simulink model "sf_elevator_old"  (R2017b)
settings: Solver=FixedStepDiscrete  StartTime=0.0  StopTime=inf  FixedStep=0.01  RelTol=1e-3  EnableMultiTasking=on
InitFcn:
  | allCarIds = [1 2];
StartFcn:
  | sf_elevator_gui('init', 'sf_elevator_old', allCarIds);
StopFcn:
  | sf_elevator_gui('close');
CloseFcn:
  | sf_elevator_gui('close');
  | clear allCarIds;
settings Model: ExtModeAutoUpdateStatusClock=off  Creator=The MathWorks, Inc.  LastModifiedBy=The MathWorks, Inc.
settings DataIOCC: LimitDataPoints=on  SaveFormat=StructureWithTime  SignalLoggingName=sigsOut
settings OptimizationCC: ExpressionDepthLimit=2147483647  InitFltsAndDblsToZero=on  EfficientMapNaN2IntZero=off  LifeSpan=Inf
settings DebuggingCC: SaveWithParameterizedLinksMsg=none  UnderspecifiedInitializationDetection=Classic  MergeDetectMultiDrivingBlocksExec=none  MultiTaskDSMMsg=warning  MultiTaskCondExecSysMsg=none  MultiTaskRateTransMsg=warning  FcnCallInpInsideContextMsg=warning  StateNameClashWarn=warning  StrictBusMsg=None  SFUnexpectedBacktrackingDiag=warning  SFNoUnconditionalDefaultTransitionDiag=warning  SFExecutionAtInitializationDiag=none
settings HardwareCC: ProdBitPerPointer=32  ProdBitPerSizeT=32  ProdBitPerPtrDiffT=32  ProdLargestAtomicFloat=None  ProdIntDivRoundTo=Undefined  ProdEndianess=Unspecified  ProdWordSize=32  ProdHWDeviceType=32-bit Generic  TargetUnknown=on
settings ModelReferenceCC: PropagateSignalLabelsOutOfModel=off
settings SFSimCC: SFSimEcho=off  SimIntegrity=off  SimParseCustomCode=off  MATLABDynamicMemAlloc=off
settings RTWCC: SystemTargetFile=ert.tlc  TemplateMakefile=ert_default_tmf  Description=Real-Time Workshop Embedded Coder
settings CodeAppCC: IgnoreCustomStorageClasses=off  CustomSymbolStrType=$N$R$M  StateflowObjectComments=on  InternalIdentifier=Classic
settings ERTTargetCC: MultiwordLength=2048  GenerateSampleERTMain=on  ERTCustomFileTemplate=example_file_process.tlc  ConvertIfToSwitch=off  SuppressUnreachableDefaultCases=off
settings ConfigComp: CovMetricSettings=dcmtr  CovHtmlReporting=on  CovSaveCumulativeToWorkspaceVar=on  CovSaveSingleToWorkspaceVar=on  CovExternalEMLEnable=off  CovSFcnEnable=off

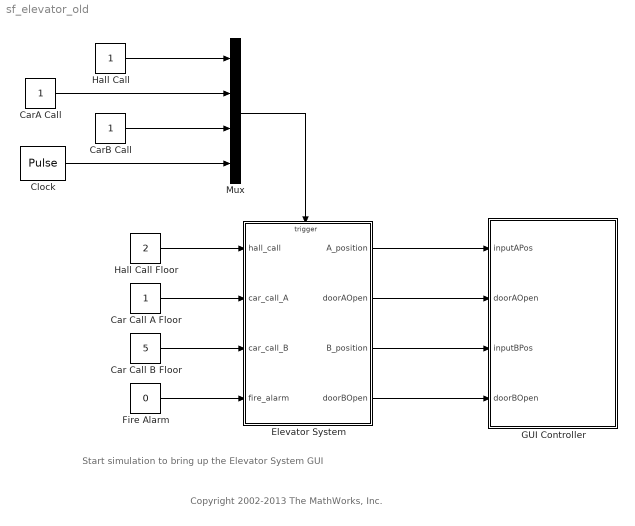
== system sf_elevator_old ==
  note: Start simulation to bring up the Elevator System GUI
  note: Copyright 2002-2013 The MathWorks, Inc.
  Car Call A Floor : Constant  OutDataTypeStr=uint8
  Car Call B Floor : Constant  Value=5  OutDataTypeStr=uint8
  CarA Call : Constant  OutDataTypeStr=double
  CarB Call : Constant  OutDataTypeStr=double
  Clock : DiscretePulseGenerator  PulseType=Time based  PulseWidth=50
  Elevator System : Stateflow chart  TreatAsAtomicUnit=on
  Fire Alarm : Constant  Value=0  OutDataTypeStr=uint8
  GUI Controller : Stateflow chart  TreatAsAtomicUnit=on
  Hall Call : Constant  OutDataTypeStr=double
  Hall Call Floor : Constant  Value=2  OutDataTypeStr=uint8
  Mux : Mux
  wires:
  Hall Call Floor/1 -> Elevator System/1(hall_call)
  Car Call A Floor/1 -> Elevator System/2(car_call_A)
  Car Call B Floor/1 -> Elevator System/3(car_call_B)
  Fire Alarm/1 -> Elevator System/4(fire_alarm)
  Hall Call/1 -> Mux/1
  CarA Call/1 -> Mux/2
  CarB Call/1 -> Mux/3
  Clock/1 -> Mux/4
  Mux/1 -> Elevator System/Trigger
  Elevator System/1(A_position) -> GUI Controller/1(inputAPos)
  Elevator System/2(doorAOpen) -> GUI Controller/2(doorAOpen)
  Elevator System/3(B_position) -> GUI Controller/3(inputBPos)
  Elevator System/4(doorBOpen) -> GUI Controller/4(doorBOpen)

== stateflow chart sf_elevator_old/Elevator System ==
  state Elevator_Manager [parallel]
    du: A_position = Elevator_A.get_position();
    B_position = Elevator_B.get_position();
    settings: executionOrder=1
    state process_hall_call() [function]
      (default) -> (junction 1685)
      (junction 1685) -> (junction 1687) : {
          | /* 'INIT':Initialization */
          | request_floor = hall_call_queue[0];
          | }
      (junction 1687) -> (junction 1689) : {
          | /* Fire alarm is on */
          | fire_alarm_on = (fire_alarm);
          | }
      (junction 1689) -> (junction 1691) : {
          | /* There is outstanding request */
          | request_outstanding = (request_floor > 0);
          | }
      (junction 1691) -> (junction 1693) : {
          | /* Elevator A is idle */
          | elevator_A_idle = (Elevator_A.get_status() == IDLE);
          | }
      (junction 1693) -> (junction 1695) : {
          | /* Elevator B is idle */
          | elevator_B_idle = (Elevator_B.get_status() == IDLE);
          | }
      (junction 1695) -> (junction 1697) : {
          | /* Elevator A is closer to request */
          | elevator_A_closer = (fabs(Elevator_A.get_position() - request_floor) <= fabs(Elevator_B.get_position() - request_floor));
          | }
      (junction 1697) -> (junction 1699) [order 1] : [fire_alarm_on]
      (junction 1699) -> (junction 1701) : {
          | /* 'EMR':Emergency */
          | Elevator_A.register(floor(Elevator_A.get_position()+Elevator_A.get_direction()/2));
          | Elevator_B.register(floor(Elevator_B.get_position()+Elevator_B.get_direction()/2));
          | }
      (junction 1697) -> (junction 1703) [order 2]
      (junction 1703) -> (junction 1705) [order 1] : [!request_outstanding]
      (junction 1705) -> (junction 1707) : {
          | /* 'NONE':Both elevators are busy or no request present */
          |
          | }
      (junction 1703) -> (junction 1709) [order 2]
      (junction 1709) -> (junction 1711) [order 1] : [!elevator_A_idle && !elevator_B_idle]
      (junction 1711) -> (junction 1713) : {
          | /* 'NONE':Both elevators are busy or no request present */
          |
          | }
      (junction 1709) -> (junction 1715) [order 2]
      (junction 1715) -> (junction 1717) [order 1] : [elevator_A_idle && !elevator_B_idle]
      (junction 1717) -> (junction 1719) : {
          | /* 'A':Elevator A should respond to request */
          | Elevator_A.enqueue(request_floor);
          | dequeue(request_floor);
          | }
      (junction 1715) -> (junction 1721) [order 2]
      (junction 1721) -> (junction 1723) [order 1] : [!elevator_A_idle && elevator_B_idle]
      (junction 1723) -> (junction 1725) : {
          | /* 'B':Elevator B should respond to request */
          | Elevator_B.enqueue(request_floor);
          | dequeue(request_floor);
          | }
      (junction 1721) -> (junction 1727) [order 2]
      (junction 1727) -> (junction 1729) [order 1] : [elevator_A_idle && elevator_B_idle && elevator_A_closer]
      (junction 1729) -> (junction 1731) : {
          | /* 'A':Elevator A should respond to request */
          | Elevator_A.enqueue(request_floor);
          | dequeue(request_floor);
          | }
      (junction 1727) -> (junction 1733) [order 2]
      (junction 1733) -> (junction 1735) [order 1] : [elevator_A_idle && elevator_B_idle && !elevator_A_closer]
      (junction 1735) -> (junction 1737) : {
          | /* 'B':Elevator B should respond to request */
          | Elevator_B.enqueue(request_floor);
          | dequeue(request_floor);
          | }
      (junction 1733) -> (junction 1739) [order 2]
    state ans = exists_in_queue(floor) [function]
      (default) -> (junction 304) : {i=0;}
      (junction 304) -> (junction 304) [order 1] : [hall_call_queue[i] > 0 && ...
          | i<NUM_FLOOR && ...
          | hall_call_queue[i] != floor]{i++;}
      (junction 304) -> (junction 303) [order 2]
      (junction 303) -> (junction 302) [order 1] : [i >= NUM_FLOOR || hall_call_queue[i] == 0]{ans = 0;}
      (junction 303) -> (junction 301) [order 2] : {ans = i+1;}
    state register(hall_call_floor) [function]
      (default) -> (junction 269) : {enqueue(hall_call_floor);
          | hall_call_status[hall_call_floor] = 1;}
    state deregister(hall_call_floor) [function]
      (default) -> (junction 272) : {dequeue(hall_call_floor);
          | hall_call_status[hall_call_floor] = 0;}
    state enqueue(hall_call_floor) [function]
      (default) -> (junction 217)
      (junction 217) -> (junction 216) [order 1] : [hall_call_status[hall_call_floor] != 0]
      (junction 217) -> (junction 234) [order 2] : {i = 0;}
      (junction 234) -> (junction 233) [order 1] : [hall_call_queue[i] == hall_call_floor]
      (junction 234) -> (junction 234) [order 2] : [hall_call_queue[i] > 0 && i<NUM_FLOOR]{i++;}
      (junction 234) -> (junction 232) [order 3]
      (junction 232) -> (junction 227) [order 1] : [i >= NUM_FLOOR]
      (junction 232) -> (junction 228) [order 2] : {hall_call_queue[i] = hall_call_floor;}
    state dequeue(hall_call_floor) [function]
      (default) -> (junction 231) : {i=0;}
      (junction 231) -> (junction 231) [order 1] : [hall_call_queue[i] > 0 && ...
          | i<NUM_FLOOR && ...
          | hall_call_queue[i] != hall_call_floor]{i++;}
      (junction 231) -> (junction 212) [order 2]
      (junction 212) -> (junction 211) [order 1] : [i >= NUM_FLOOR || hall_call_queue[i] == 0]
      (junction 212) -> (junction 206) [order 2]
      (junction 206) -> (junction 230) : {hall_call_queue[i] = hall_call_queue[i+1]; i++;}
      (junction 230) -> (junction 206) [order 1] : [i < NUM_FLOOR]
      (junction 230) -> (junction 274) [order 2]
    Elevator_Manager -> (junction 229) [order 1] : HALL_CALL{register(hall_call);}
    Elevator_Manager -> (junction 1430) [order 2] : CLOCK {process_hall_call();}
  state Elevator_B [parallel]
    settings: executionOrder=3
    state PickUpDropOff
      en: Elevator_Manager.deregister(cur_floor);
      deregister(cur_floor);
      direction = MOVE_IDLE;
      doorBOpen = 1;
      du: Elevator_Manager.deregister(cur_floor);
      deregister(cur_floor);
      ex: doorBOpen = 0;
      state Stopped
      Elevator_B.PickUpDropOff.Stopped -> Elevator_B.PickUpDropOff.Stopped [order 2] : [fire_alarm]{status = EMERG;}
          | /* Resets the timeout counter */
    state Idle
      en: status = IDLE;
      ex: status = BUSY;
    state MoveToTask
      du: move_to(task_queue[0]);
    state move_to(destination) [function]
      (default) -> (junction 1615)
      (junction 1615) -> (junction 1617) : {
          | /* Move up */
          | move_up = (destination - position > ERR_TOR);
          | }
      (junction 1617) -> (junction 1619) : {
          | /* Move down */
          | move_down = (position - destination > ERR_TOR);
          | }
      (junction 1619) -> (junction 1621) [order 1] : [move_up && !move_down]
      (junction 1621) -> (junction 1623) : {
          | /* Move up */
          | position = position + VELOCITY;
          | direction = MOVE_UP;
          | }
      (junction 1619) -> (junction 1625) [order 2]
      (junction 1625) -> (junction 1627) [order 1] : [!move_up && move_down]
      (junction 1627) -> (junction 1629) : {
          | /* Move down */
          | position = position - VELOCITY;
          | direction = MOVE_DOWN;
          | }
      (junction 1625) -> (junction 1631) [order 2]
    state ans = should_stop [function]
      (default) -> (junction 1638)
      (junction 1638) -> (junction 1640) : {
          | /* 'INIT':Initialization */
          | cur_floor = ml_round(position);
          | }
      (junction 1640) -> (junction 1642) : {
          | /* Arrived destination */
          | at_destination = (fabs(position - task_queue[0]) < ERR_TOR);
          | }
      (junction 1642) -> (junction 1644) : {
          | /* Arrived a floor */
          | at_a_floor = (fabs(position - cur_floor) < ERR_TOR);
          | }
      (junction 1644) -> (junction 1646) : {
          | /* There is car call to stop at this floor */
          | request_from_car = (car_call_status[cur_floor]);
          | }
      (junction 1646) -> (junction 1648) : {
          | /* There is hall call from this floor */
          | request_from_hall = (Elevator_Manager.hall_call_status[cur_floor]);
          | }
      (junction 1648) -> (junction 1650) : {
          | /* This hall call is still outstanding in queue */
          | this_hall_call_outstanding = (Elevator_Manager.exists_in_queue(cur_floor));
          | }
      (junction 1650) -> (junction 1652) [order 1] : [at_destination]
      (junction 1652) -> (junction 1654) : {
          | /* 'S':Should stop at this floor */
          | position = cur_floor; /* Adjust position */
          | ans = 1;
          | }
      (junction 1650) -> (junction 1656) [order 2]
      (junction 1656) -> (junction 1658) [order 1] : [!at_a_floor]
      (junction 1658) -> (junction 1660) : {
          | /* 'C':Should not stop, continue */
          | ans = 0;
          | }
      (junction 1656) -> (junction 1662) [order 2]
      (junction 1662) -> (junction 1664) [order 1] : [request_from_car]
      (junction 1664) -> (junction 1666) : {
          | /* 'S':Should stop at this floor */
          | position = cur_floor; /* Adjust position */
          | ans = 1;
          | }
      (junction 1662) -> (junction 1668) [order 2]
      (junction 1668) -> (junction 1670) [order 1] : [request_from_hall && this_hall_call_outstanding]
      (junction 1670) -> (junction 1672) : {
          | /* 'S':Should stop at this floor */
          | position = cur_floor; /* Adjust position */
          | ans = 1;
          | }
      (junction 1668) -> (junction 1674) [order 2]
      (junction 1674) -> (junction 1676) : /* Default */
      (junction 1676) -> (junction 1678) : {
          | /* 'C':Should not stop, continue */
          | ans = 0;
          | }
    state dir = get_direction [function]
      (default) -> (junction 947) : {dir = direction;}
    state register(car_call_floor) [function]
      (default) -> (junction 951) : {enqueue(car_call_floor);
          | car_call_status[car_call_floor] = 1;}
    state enqueue(task_floor) [function]
      (default) -> (junction 956)
      (junction 956) -> (junction 957) [order 1] : [car_call_status[task_floor] != 0]
      (junction 956) -> (junction 959) [order 2] : {i = 0;}
      (junction 959) -> (junction 958) [order 1] : [task_queue[i] == task_floor]
      (junction 959) -> (junction 959) [order 2] : [task_queue[i] > 0 && i<NUM_FLOOR]{i++;}
      (junction 959) -> (junction 960) [order 3]
      (junction 960) -> (junction 961) [order 1] : [i >= NUM_FLOOR]
      (junction 960) -> (junction 962) [order 2] : {task_queue[i] = task_floor;}
    state pos = get_position [function]
      (default) -> (junction 973) : {pos = position;}
    state deregister(car_call_floor) [function]
      (default) -> (junction 977) : {dequeue(car_call_floor);
          | car_call_status[car_call_floor] = 0;}
    state stat = get_status [function]
      (default) -> (junction 981) : {stat = status;}
    state dequeue(task_floor) [function]
      (default) -> (junction 986) : {i=0;}
      (junction 986) -> (junction 986) [order 1] : [task_queue[i] > 0 && ...
          | i<NUM_FLOOR && ...
          | task_queue[i] != task_floor]{i++;}
      (junction 986) -> (junction 987) [order 2]
      (junction 987) -> (junction 988) [order 1] : [i >= NUM_FLOOR || task_queue[i] == 0]
      (junction 987) -> (junction 989) [order 2]
      (junction 989) -> (junction 990) : {task_queue[i] = task_queue[i+1]; i++;}
      (junction 990) -> (junction 989) [order 1] : [i < NUM_FLOOR]
      (junction 990) -> (junction 991) [order 2]
    Elevator_B -> (junction 1744) : CAR_CALL_B{Elevator_B.register(car_call_B);}
    (default) -> Elevator_B.Idle : {doorBOpen = 0;}
    (junction 862) -> Elevator_B.Idle [order 2]
    Elevator_B.PickUpDropOff.Stopped -> (junction 862) [order 1] : after(TIME_OUT, CLOCK)
    (junction 862) -> Elevator_B.MoveToTask [order 1] : [task_queue[0]]
    Elevator_B.Idle -> Elevator_B.MoveToTask : [task_queue[0]]
    Elevator_B.MoveToTask -> Elevator_B.PickUpDropOff : [should_stop()]
  state Elevator_A [parallel]
    settings: executionOrder=2
    state PickUpDropOff
      en: Elevator_Manager.deregister(cur_floor);
      deregister(cur_floor);
      direction = MOVE_IDLE;
      doorAOpen = 1;
      du: Elevator_Manager.deregister(cur_floor);
      deregister(cur_floor);
      ex: doorAOpen = 0;
      state Stopped
      Elevator_A.PickUpDropOff.Stopped -> Elevator_A.PickUpDropOff.Stopped [order 2] : [fire_alarm]{status = EMERG;}
          | /* Resets the timeout counter */
    state Idle
      en: status = IDLE;
      ex: status = BUSY;
    state MoveToTask
      du: move_to(task_queue[0]);
    state move_to(destination) [function]
      (default) -> (junction 1548)
      (junction 1548) -> (junction 1550) : {
          | /* Move up */
          | move_up = (destination - position > ERR_TOR);
          | }
      (junction 1550) -> (junction 1552) : {
          | /* Move down */
          | move_down = (position - destination > ERR_TOR);
          | }
      (junction 1552) -> (junction 1554) [order 1] : [move_up && !move_down]
      (junction 1554) -> (junction 1556) : {
          | /* Move up */
          | position = position + VELOCITY;
          | direction = MOVE_UP;
          | }
      (junction 1552) -> (junction 1558) [order 2]
      (junction 1558) -> (junction 1560) [order 1] : [!move_up && move_down]
      (junction 1560) -> (junction 1562) : {
          | /* Move down */
          | position = position - VELOCITY;
          | direction = MOVE_DOWN;
          | }
      (junction 1558) -> (junction 1564) [order 2]
    state ans = should_stop() [function]
      (default) -> (junction 1571)
      (junction 1571) -> (junction 1573) : {
          | /* 'INIT':Initialization */
          | cur_floor = ml_round(position);
          | }
      (junction 1573) -> (junction 1575) : {
          | /* Arrived destination */
          | at_destination = (fabs(position - task_queue[0]) < ERR_TOR);
          | }
      (junction 1575) -> (junction 1577) : {
          | /* Arrived a floor */
          | at_a_floor = (fabs(position - cur_floor) < ERR_TOR);
          | }
      (junction 1577) -> (junction 1579) : {
          | /* There is car call to stop at this floor */
          | request_from_car = (car_call_status[cur_floor]);
          | }
      (junction 1579) -> (junction 1581) : {
          | /* There is hall call from this floor */
          | request_from_hall = (Elevator_Manager.hall_call_status[cur_floor]);
          | }
      (junction 1581) -> (junction 1583) : {
          | /* This hall call is still outstanding in queue */
          | this_hall_call_outstanding = (Elevator_Manager.exists_in_queue(cur_floor));
          | }
      (junction 1583) -> (junction 1585) [order 1] : [at_destination]
      (junction 1585) -> (junction 1587) : {
          | /* 'S':Should stop at this floor */
          | position = cur_floor; /* Adjust position */
          | ans = 1;
          | }
      (junction 1583) -> (junction 1589) [order 2]
      (junction 1589) -> (junction 1591) [order 1] : [!at_a_floor]
      (junction 1591) -> (junction 1593) : {
          | /* 'C':Should not stop, continue */
          | ans = 0;
          | }
      (junction 1589) -> (junction 1595) [order 2]
      (junction 1595) -> (junction 1597) [order 1] : [request_from_car]
      (junction 1597) -> (junction 1599) : {
          | /* 'S':Should stop at this floor */
          | position = cur_floor; /* Adjust position */
          | ans = 1;
          | }
      (junction 1595) -> (junction 1601) [order 2]
      (junction 1601) -> (junction 1603) [order 1] : [request_from_hall && this_hall_call_outstanding]
      (junction 1603) -> (junction 1605) : {
          | /* 'S':Should stop at this floor */
          | position = cur_floor; /* Adjust position */
          | ans = 1;
          | }
      (junction 1601) -> (junction 1607) [order 2]
      (junction 1607) -> (junction 1609) : /* Default */
      (junction 1609) -> (junction 1611) : {
          | /* 'C':Should not stop, continue */
          | ans = 0;
          | }
    state dir = get_direction() [function]
      (default) -> (junction 247) : {dir = direction;}
    state register(car_call_floor) [function]
      (default) -> (junction 270) : {enqueue(car_call_floor);
          | car_call_status[car_call_floor] = 1;}
    state enqueue(task_floor) [function]
      (default) -> (junction 215)
      (junction 215) -> (junction 214) [order 1] : [car_call_status[task_floor] != 0]
      (junction 215) -> (junction 225) [order 2] : {i = 0;}
      (junction 225) -> (junction 226) [order 1] : [task_queue[i] == task_floor]
      (junction 225) -> (junction 225) [order 2] : [task_queue[i] > 0 && i<NUM_FLOOR]{i++;}
      (junction 225) -> (junction 224) [order 3]
      (junction 224) -> (junction 223) [order 1] : [i >= NUM_FLOOR]
      (junction 224) -> (junction 213) [order 2] : {task_queue[i] = task_floor;}
    state pos = get_position() [function]
      (default) -> (junction 210) : {pos = position;}
    state deregister(car_call_floor) [function]
      (default) -> (junction 271) : {dequeue(car_call_floor);
          | car_call_status[car_call_floor] = 0;}
    state stat = get_status() [function]
      (default) -> (junction 209) : {stat = status;}
    state dequeue(task_floor) [function]
      (default) -> (junction 208) : {i=0;}
      (junction 208) -> (junction 208) [order 1] : [task_queue[i] > 0 && ...
          | i<NUM_FLOOR && ...
          | task_queue[i] != task_floor]{i++;}
      (junction 208) -> (junction 207) [order 2]
      (junction 207) -> (junction 235) [order 1] : [i >= NUM_FLOOR || task_queue[i] == 0]
      (junction 207) -> (junction 236) [order 2]
      (junction 236) -> (junction 218) : {task_queue[i] = task_queue[i+1]; i++;}
      (junction 218) -> (junction 236) [order 1] : [i < NUM_FLOOR]
      (junction 218) -> (junction 273) [order 2]
    Elevator_A -> (junction 1741) : CAR_CALL_A{Elevator_A.register(car_call_A);}
    (default) -> Elevator_A.Idle : {doorAOpen = 0;}
    (junction 240) -> Elevator_A.Idle [order 2]
    Elevator_A.PickUpDropOff.Stopped -> (junction 240) [order 1] : after(TIME_OUT, CLOCK)
    (junction 240) -> Elevator_A.MoveToTask [order 1] : [task_queue[0]]
    Elevator_A.Idle -> Elevator_A.MoveToTask : [task_queue[0]]
    Elevator_A.MoveToTask -> Elevator_A.PickUpDropOff : [should_stop()]
  data: request_floor temporary uint8; fire_alarm_on temporary boolean =0; request_outstanding temporary boolean =0; elevator_A_idle temporary boolean =0; elevator_B_idle temporary boolean =0; elevator_A_closer temporary boolean =0; ans function_output uint8; floor function_input uint8; i temporary uint8; hall_call_floor function_input uint8; hall_call_floor function_input uint8; hall_call_floor function_input uint8; i temporary uint8; i temporary uint8; hall_call_floor function_input uint8; hall_call_queue local uint8 size=10; hall_call_status local uint8 size=10; destination function_input double; move_up temporary boolean =0; move_down temporary boolean =0; ans function_output boolean; at_destination temporary boolean =0; at_a_floor temporary boolean =0; request_from_car temporary boolean =0; request_from_hall temporary boolean =0; this_hall_call_outstanding temporary boolean =0; dir function_output uint8; car_call_floor function_input uint8; task_floor function_input uint8; i temporary uint8; pos function_output double; car_call_floor function_input uint8; stat function_output uint8; i temporary uint8; task_floor function_input uint8; inputVal function_input double; out function_output double; position local double =1; task_queue local uint8 size=10; car_call_status local uint8 size=10; cur_floor local uint8; direction local Enum: ElevatorDirection =ElevatorDirection.MOVE_IDLE; status local Enum: ElevatorStatus =ElevatorStatus.IDLE; destination function_input double; move_up temporary boolean =0; move_down temporary boolean =0; ans function_output boolean; at_destination temporary boolean =0; at_a_floor temporary boolean =0; request_from_car temporary boolean =0; request_from_hall temporary boolean =0; this_hall_call_outstanding temporary boolean =0; dir function_output uint8; car_call_floor function_input uint8; task_floor function_input uint8; i temporary uint8; pos function_output double; car_call_floor function_input uint8; stat function_output uint8; i temporary uint8; task_floor function_input uint8; inputVal function_input double; out function_output double; status local Enum: ElevatorStatus =ElevatorStatus.IDLE; position local double =1; task_queue local uint8 size=10; car_call_status local uint8 size=10; cur_floor local uint8; direction local Enum: ElevatorDirection =ElevatorDirection.MOVE_IDLE; VELOCITY constant double =0.005; hall_call input uint8; A_position output double =1; doorAOpen output boolean; B_position output double =1; NUM_FLOOR constant uint8 =9; ERR_TOR constant double =0.001; car_call_A input uint8; car_call_B input uint8; fire_alarm input uint8; TIME_OUT constant uint32 =1000; doorBOpen output boolean
  data fire_alarm_on settings: description=Fire alarm is on
  data request_outstanding settings: description=There is outstanding request
  data elevator_A_idle settings: description=Elevator A is idle
  data elevator_B_idle settings: description=Elevator B is idle
  data elevator_A_closer settings: description=Elevator A is closer to request
  data move_up settings: description=Move up
  data move_down settings: description=Move down
  data at_destination settings: description=Arrived destination
  data at_a_floor settings: description=Arrived a floor
  data request_from_car settings: description=There is car call to stop at this floor
  data request_from_hall settings: description=There is hall call from this floor
  data this_hall_call_outstanding settings: description=This hall call is still outstanding in queue
  data move_up settings: description=Move up
  data move_down settings: description=Move down
  data at_destination settings: description=Arrived destination
  data at_a_floor settings: description=Arrived a floor
  data request_from_car settings: description=There is car call to stop at this floor
  data request_from_hall settings: description=There is hall call from this floor
  data this_hall_call_outstanding settings: description=This hall call is still outstanding in queue
  events: HALL_CALL input EITHER_EDGE_EVENT; CAR_CALL_A input EITHER_EDGE_EVENT; CAR_CALL_B input EITHER_EDGE_EVENT; CLOCK input EITHER_EDGE_EVENT
  function out = ml_round(inputVal):
    | function out = ml_round(inputVal)
    | 
    | out = round(inputVal);
  function out = ml_round(inputVal):
    | function out = ml_round(inputVal)
    | 
    | out = round(inputVal);

== stateflow chart sf_elevator_old/GUI Controller ==
  state CarA_Controller [parallel]
    settings: executionOrder=1
    state close_door [function]
      (default) -> (junction 203) : {ml.sf_elevator_gui('close_door', allCarIds[0]);}
    state open_door [function]
      (default) -> (junction 206) : {ml.sf_elevator_gui('open_door', allCarIds[0]);}
    state move(pos) [function]
      (default) -> (junction 210) : {ml.sf_elevator_gui('move_car', allCarIds[0], pos);}
    state deactivate_hall_button(pos) [function]
      (default) -> (junction 231) : {floorNum = get_floor_number(pos);
          | ml.sf_elevator_gui('deactivate','hall', floorNum);}
    state deactivate_car_button(pos) [function]
      (default) -> (junction 219) : {floorNum = get_floor_number(pos);
          | ml.sf_elevator_gui('deactivate',allCarIds[0], floorNum);}
    state floorNumber = get_floor_number(pos) [function]
      (default) -> (junction 224) : {floorNumber = ml.round(pos);}
    CarA_Controller -> (junction 175)
    (junction 175) -> (junction 176) [order 1] : [hasChanged(inputAPos)]
    (junction 175) -> (junction 177) [order 2]
    (junction 176) -> (junction 178) : {move(inputAPos);}
    (junction 178) -> (junction 177)
    (junction 177) -> (junction 179)
    (junction 179) -> (junction 180) [order 1] : [hasChanged(doorAOpen)]
    (junction 179) -> (junction 183) [order 2]
    (junction 180) -> (junction 181)
    (junction 181) -> (junction 182) [order 1] : [doorAOpen]
    (junction 181) -> (junction 184) [order 2] : {close_door();}
    (junction 182) -> (junction 185) : {open_door();}
    (junction 184) -> (junction 183) : {deactivate_hall_button(inputAPos);
        |  deactivate_car_button(inputAPos);}
    (junction 185) -> (junction 184)
    (junction 183) -> (junction 186)
  state CarB_Controller [parallel]
    settings: executionOrder=2
    state close_door [function]
      (default) -> (junction 263) : {ml.sf_elevator_gui('close_door', allCarIds[1]);}
    state open_door [function]
      (default) -> (junction 288) : {ml.sf_elevator_gui('open_door', allCarIds[1]);}
    state move(pos) [function]
      (default) -> (junction 270) : {ml.sf_elevator_gui('move_car', allCarIds[1], pos);}
    state deactivate_hall_button(pos) [function]
      (default) -> (junction 286) : {floorNum = get_floor_number(pos);
          | ml.sf_elevator_gui('deactivate','hall', floorNum);}
    state deactivate_car_button(pos) [function]
      (default) -> (junction 279) : {floorNum = get_floor_number(pos);
          | ml.sf_elevator_gui('deactivate',allCarIds[1], floorNum);}
    state floorNumber = get_floor_number(pos) [function]
      (default) -> (junction 284) : {floorNumber = ml.round(pos);}
    CarB_Controller -> (junction 235)
    (junction 235) -> (junction 236) [order 1] : [hasChanged(inputBPos)]
    (junction 235) -> (junction 237) [order 2]
    (junction 236) -> (junction 238) : {move(inputBPos);}
    (junction 238) -> (junction 237)
    (junction 237) -> (junction 239)
    (junction 239) -> (junction 240) [order 1] : [hasChanged(doorBOpen)]
    (junction 239) -> (junction 243) [order 2]
    (junction 240) -> (junction 241)
    (junction 241) -> (junction 242) [order 1] : [doorBOpen]
    (junction 241) -> (junction 244) [order 2] : {close_door();}
    (junction 242) -> (junction 245) : {open_door();}
    (junction 244) -> (junction 243) : {deactivate_hall_button(inputBPos);
        |  deactivate_car_button(inputBPos);}
    (junction 245) -> (junction 244)
    (junction 243) -> (junction 246)
  data: pos function_input double; pos function_input double; floorNum temporary double; pos function_input double; floorNum temporary double; pos function_input double; floorNumber function_output double; pos function_input double; pos function_input double; floorNum temporary double; pos function_input double; floorNum temporary double; pos function_input double; floorNumber function_output double; inputAPos input; doorAOpen input; inputBPos input; doorBOpen input; allCarIds parameter uint8 size=2
